simulink subsystem "EncodersAJz"  (R2023b)
settings: Solver=VariableStepAuto  StartTime=0.0  StopTime=10.0  RelTol=1e-3
libraries: arduinosensorlib x2, simulink x1
settings Model: Creator=jaime  LastModifiedBy=jaime

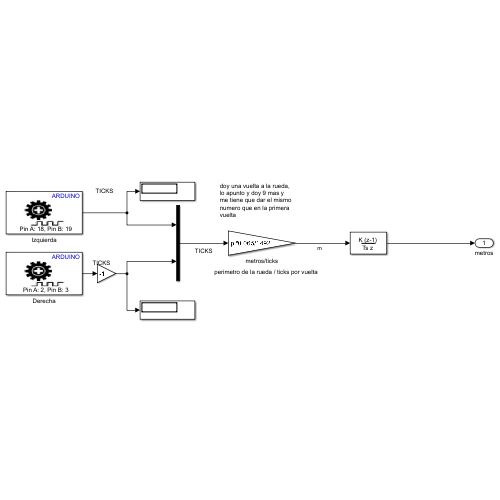
[thumbnail: Simulink's stored preview of the top-level diagram]
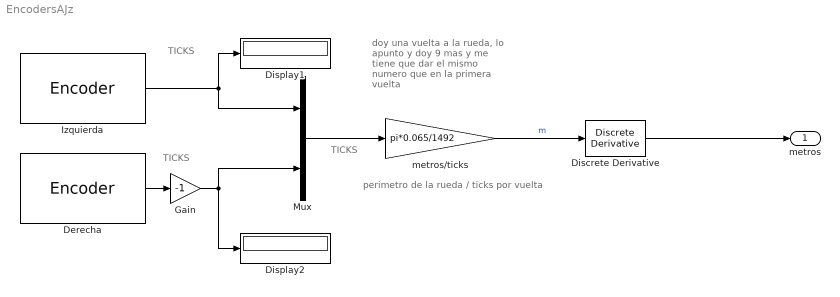
== system EncodersAJz ==
  note: TICKS
  note: TICKS
  note: TICKS
  note: perimetro de la rueda / ticks por vuelta
  note: doy una vuelta a la rueda, lo apunto y doy 9 mas y me tiene que dar el mismo numero que en la primera vuelta
  Derecha : arduinosensorlib/Encoder  InputA=2  InputB=3  Mode=No reset  SampleTime=-1
  Discrete Derivative : simulink/Discrete/Discrete Derivative  gainval=1.0  ICPrevScaledInput=0.0  OutMin=[]  OutMax=[]  OutDataType=fixdt(1, 16)  OutScaling=2^-10  DoSatur=off
  Display1 : Display
  Display2 : Display
  Gain : Gain  Gain=-1  OutDataTypeStr=int32
  Izquierda : arduinosensorlib/Encoder  InputA=18  InputB=19  Mode=No reset  SampleTime=-1
  Mux : Mux  Inputs=2
  metros/ticks : Gain  Gain=pi*0.065/1492  OutDataTypeStr=double
  metros : Outport
  wires:
  Derecha/1 -> Gain/1
  Mux/1 -> metros/ticks/1
  Izquierda/1 -> Display1/1, Mux/1
  Gain/1 -> Display2/1, Mux/2
  metros/ticks/1 -> Discrete Derivative/1  "m"
  Discrete Derivative/1 -> metros/1
